simulink model "psbdynamicload"  (Simulink 6.0)
settings: Solver=ode23tb  SolverMode=SingleTasking  StartTime=0.0  StopTime=1.4  FixedStep=Ts  RelTol=1e-3
InitFcn:
  | powericon('psbinitsys',bdroot);
libraries: powerlib2 x7, powerlib_extras x2
settings Model: Creator=sybille  LastModifiedBy=batserve  ExtModeTrigMode=oneshot  ExtModeArmWhenConnect=off  ExtModeAutoUpdateStatusClock=off  ProdHWDeviceType=Specified
settings DataIOCC: LimitDataPoints=off  SaveOutput=off  SaveTime=off  SignalLoggingName=sigsOut
settings OptimizationCC: BooleanDataType=off
settings DebuggingCC: CheckExecutionContextPreStartOutputMsg=on  CheckExecutionContextRuntimeOutputMsg=on  SolverPrmCheckMsg=none
settings HardwareCC: ProdBitPerShort=32  ProdBitPerInt=16  ProdHWDeviceType=Specified  TargetUnknown=on

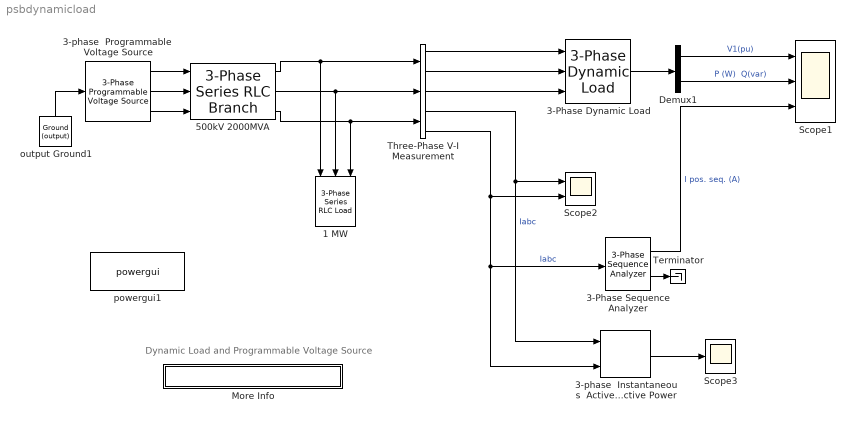
== system psbdynamicload ==
  note: Dynamic Load and Programmable Voltage Source
  1 MW : powerlib2/Elements/3-Phase Series RLC Load  Orientation=down  Vpp=500e3  fn=60  P3=1e6  QL3=0  QC3=0
  3-Phase Dynamic Load : powerlib2/Elements/3-Phase Dynamic Load  Vfnom=[ 500e3 60 ]  PQ_0=[5e+007 2.5e+007]  V0=[0.98441 -1.41063]  PQext=off  n="[1  1]"  Tpq="[0  0  0  0]"  Vmin=0.7  LoadFlowParameters=[4 50000000 0 0 25000000]
  3-Phase Sequence Analyzer : powerlib_extras/Measurements/3-Phase Sequence Analyzer  f1=60  n=1  seq=Positive
  3-phase  Instantaneous  Active & Reactive Power : powerlib_extras/Measurements/3-phase  Instantaneous  Active & Reactive Power  AncestorBlock=|
      | powerlib_extras/Discrete
      | Measurements/3-phase
      | Instantaneous 
      | Active and Reactive
      | Power Computation
  3-phase  Programmable  Voltage Source : powerlib2/Electrical Sources/3-Phase  Programmable  Voltage Source  Par_Vps_LLrms="[500e3 0  60]"  VariationEntity=Amplitude  VariationType=Modulation  VariationStep=-0.5  VariationRate=10  VariationMag=0.5  VariationFreq=1  Par_Timing_Variation=[0.2 1.2]  SinglePhase=off  Yampli=[1 0.8 1.2 1.0]  Xtime=[0 0.1 0.15 0.2]  HarmonicGeneration=off  Par_HarmoA_pu=[3 0.2 -25 0]  Par_HarmoB_pu="[2 0.15  35 2]"  Par_Timing_Harmo="[0.05  3]"
  500kV 2000MVA : powerlib2/Elements/3-Phase Series RLC Branch   R=500^2/2000/10  L=500^2/2000/377  C=inf
  Demux1 : Demux  Outputs=[1 2]
  More Info : Subsystem
      mask Display: disp('? : Double click here for more info')
  Scope1 : Scope  NumInputPorts=3
      settings: TimeRange=1.4  YMin=0.4000000000000001~5000000~62.5  YMax=1.5~80000000~95
  Scope2 : Scope  NumInputPorts=2
      settings: TimeRange=1.4  YMin=-1000000~-100  YMax=1000000~100
  Scope3 : Scope
      settings: TimeRange=1.4  YMin=0  YMax=80000000  SaveName=ScopeData3
  Terminator : Terminator
  Three-Phase V-I Measurement : powerlib2/Measurements/Three-Phase V-I Measurement  Tag=PoWeRsYsTeMmEaSuReMeNt  VChoice=phase-to-ground  ualv=off  labelV=V1  Vpu=off  Vbase=500e3  IChoice=yes  ualc=off  labelC=I1  Ppu=off  Pbase=100e6  OutputType=Magnitude  PhasorSimulation=off  PSBequivalent=1  PSBOutputType=11100
  output Ground1 : powerlib2/Connectors/Ground (output)  Tag=PoWeRsYsTeMbLoCk  Orientation=up  PSBOutputType=1
  powergui1 : powerlib2/powergui  Frange=[0:2:500]  Ylog=off  Xlog=off  save=off  variable=ZData  ZoomFFT=on  StartTime=0.0  cycles=1  DisplayStyle=off  fundamental=60  FreqAxis=off  MaxFrequency=1000  frequencyindice=60  frequencyindicesteady=1  RmsSteady=2  display=off  Ts=0  methode=off  frequency=60  echomessages=off
  wires:
  Three-Phase V-I Measurement/5 -> Scope2/2, 3-Phase Sequence Analyzer/1, 3-phase  Instantaneous  Active & Reactive Power/2  "Iabc"
  Three-Phase V-I Measurement/4 -> Scope2/1, 3-phase  Instantaneous  Active & Reactive Power/1  "Iabc"
  500kV 2000MVA/1 -> 1 MW/1, Three-Phase V-I Measurement/1
  500kV 2000MVA/2 -> 1 MW/2, Three-Phase V-I Measurement/2
  500kV 2000MVA/3 -> 1 MW/3, Three-Phase V-I Measurement/3
  Three-Phase V-I Measurement/1 -> 3-Phase Dynamic Load/1
  Three-Phase V-I Measurement/2 -> 3-Phase Dynamic Load/2
  Three-Phase V-I Measurement/3 -> 3-Phase Dynamic Load/3
  3-Phase Dynamic Load/1 -> Demux1/1
  Demux1/1 -> Scope1/1  "V1(pu)"
  3-phase  Instantaneous  Active & Reactive Power/1 -> Scope3/1
  3-phase  Programmable  Voltage Source/1 -> 500kV 2000MVA/1
  3-phase  Programmable  Voltage Source/2 -> 500kV 2000MVA/2
  3-phase  Programmable  Voltage Source/3 -> 500kV 2000MVA/3
  output Ground1/1 -> 3-phase  Programmable  Voltage Source/1
  3-Phase Sequence Analyzer/1 -> Scope1/3  "I pos. seq. (A)"
  Demux1/2 -> Scope1/2  "P (W)  Q(var)"
  3-Phase Sequence Analyzer/2 -> Terminator/1

== system psbdynamicload/More Info ==
  note: G. Sybille (Hydro-Quebec)
  note: Start the simulation and observe load voltage, P&Q powers  and current on Scope1. Observe that  simulation starts in steady state. At t = 0.2 s , when voltage
      | modulation is initiated, P and Q start to increase (trace 2), but, as np and nq are set to 1, the load current  (trace 3) stays constant.. When voltage falls below 0.7 pu
      | the load behaves as a constant impedance. Therefore load current follows this voltage variation.
      | Observe on Scope2 variations of instantaneous voltages and currents. Also, notice that computed Pand Q  displayed on Scope3 are the same as  P and Q internal
      | signals returned by the Dynamic Load measurement output.
  note: A dynamic load is connected on a  500 kV, 60 Hz  power network . The network is simulated by its Thevenin equivalent (voltage source behind a R-L impedance
      | corresponding to a 3-phase short circuit level of 2000 MVA). The source internal voltage is modulated in order  to simulate voltage variation during a power swing.
      | As the dymamic load is a  nonlinear model simulated by current sources, it cannot be connected to an inductive network (R-L in series).
      | Therefore, a small resistive load (1 MW) has been added in parallel with the dynamic load.
      |
      | The dynamic load power is a function of its terminal positive-sequence voltage V. Open the Dynamic Load menu and notice that both exponents np and nq
      | are set to 1 and that the specified minimum voltage Vmin is 0.7 pu . It means that the load active power P and reactive power Q are defined by the following equations:
      |
      |       If V > Vmin
      |             P = Po*(V/Vo);    Q = Qo*(V/Vo)
      |       If V < Vmin
      |             P = Po*(V/Vo)^2;   Q = Qo*(V/Vo)^2
      |
      | In other words, as long as voltage is higher than 0.7 pu, the load current is constant. When voltage falls below 0.7 pu the load behaves as a constant impedance.
      |
      | In order to demonstrate the variation of P and Q as function of voltage, the source internal voltage is controlled by the 3-Phase Programmable Voltage Source block.
      | Open the source menu and notice that the specified type of amplitude variation is a sinusoidal modulation (Amplitude of the modulation = 0.5 pu,
      | Frequency of the modulation = 1 Hz). Therefore, the source positive-sequence voltage varies between 0.5 pu and 1.5 pu.
      | The initial source voltage is 1 pu. Modulation starts at t = 0.2 s and stops after 1 cycle at t = 1.2 s.
      |
      | A 3-Phase Sequence Analyzer block (from the Extras/Measurement library), is used to monitor the positive-sequence component of load current.
      | Another block from from the Extras/Measurement library is used to compute the load active- and reactive powers.
  note: Demonstration
  note: Circuit Description
  note: This example illustrates use of the 3-Phase Dynamic Load and 3-Phase Programmable Voltage Source blocks
  note: 1. Initializing the dynamic load
  note: In order to start the simulation in steady-state you have to specify the correct initial voltage Vo  (magnitude and phase) corresponding to desired Po and Qo
      | values. You will now use the 'Load Flow' utility to find this voltage and initialize the dynamic load.
      |
      | Open the Powergui and select 'Load Flow and Machine Initialization' .  Specify the desired active power and reactive powers for the Dynamic Load (50 MW, 25 Mvar):
      |        Active Power = 50e6  Reactive Power = 25e6.
      |
      | Then press the 'Update Load Flow' button.Once the load flow has been solved the phasors of AB and BC machine voltages as well as the currents flowing into
      | of phases A and B are updated. The phase-neutral load voltage Uan is also displayed: ( 0.9844 pu - 1.41 degrees).
      | If you now open the Dynamic Load dialog box you will notice that the values of Po, Qo and  Vo have been updated.
  note: 2. Simulating the voltage swing
